simulink model "MAS"  (R2023a)
settings: Solver=FixedStepAuto  StartTime=0.0  StopTime=1  FixedStep=1e-6  RelTol=1e-5
values from neighbouring files (symbols this model uses):
  A_ob_w = [0, 0, 0, Msr*Rr/(rau*Ls*Lr) ... (first row only)    [main.m]
  A_observateur = [-Rsr/(rau*Ls), 0, Msr*Rr/(rau*Ls*Lr^2), 0 ... (first row only)    [main.m]
  abc_alpha_beta = sqrt(2/3) * [1, -1/2, -1/2 ... (first row only)    [main.m]
  B_observateur = [1/(rau*Ls),0 ... (first row only)    [main.m]
  Flux_1 = 1/(Msr^2 - Ls * Lr )  * [Rs*Lr, 0, -Rs*Msr, 0 ... (first row only)    [main.m]
  Flux_2 = 1/(Msr^2 - Ls * Lr )  * [0, 0, 0, 0 ... (first row only)    [main.m]
  frot = 0.01    [main.m]
  In = 8.3    [main.m]
  Inv_abc_alpha_beta = inv(abc_alpha_beta)    [main.m]
  Inv_Phi_Courant = inv(Phi_Courant)    [main.m]
  J = 0.025    [main.m]
  K_observateur = [-Rs/Ls-2*Pole, 0 ... (first row only)    [main.m]
  ki_reg_flux = K_reg_flux/T_reg_flux    (= 325705.222612)    [main.m]
  ki_reg_vitesse = K_reg_vitesse    (= 0.24)    [main.m]
  kid = ki/Ti    (= 11257.7319588)    [main.m]
  kiq = ki/Ti    (= 11257.7319588)    [main.m]
  kp_reg_flux = K_reg_flux    (= 179.885332059)    [main.m]
  kp_reg_vitesse = K_reg_vitesse/T_reg_vitesse    (= 0.625)    [main.m]
  kpd = ki    (= 19.9033319163)    [main.m]
  Kpi = ws*20    (= 6283.18530718)    [main.m]
  kpq = ki    (= 19.9033319163)    [main.m]
  Lr = 0.194    [main.m]
  Ls = 0.182    [main.m]
  Msr = 0.182    [main.m]
  onduleur = V_MLI/3*[2,-1,-1 ... (first row only)    [main.m]
  p = 2    [main.m]
  Pole = 1    [main.m]
  Rr = 1.15    [main.m]
  sigma = 1-Msr^2/(Ls*Lr)    (= 0.0618556701031)    [main.m]
  T_charge = 0    [main.m]
  T_MLI = 1/F_MLI    (= 0.0001)    [main.m]
  Tin = sqrt(10)/Kpi    [main.m]
  V_MLI = 540    [main.m]
  Vn = 220    [main.m]
  ws = 2*pi*Fn    (= 314.159265359)    [main.m]
libraries: hdlsllib x5, simulink_extras x4, simulink x1
settings Model: SimulationMode=accelerator  Creator=philippecasteres  LastModifiedBy=philippecasteres
settings SolverCC: ZeroCrossAlgorithm=Adaptive
settings DebuggingCC: IgnoredZcDiagnostic=none

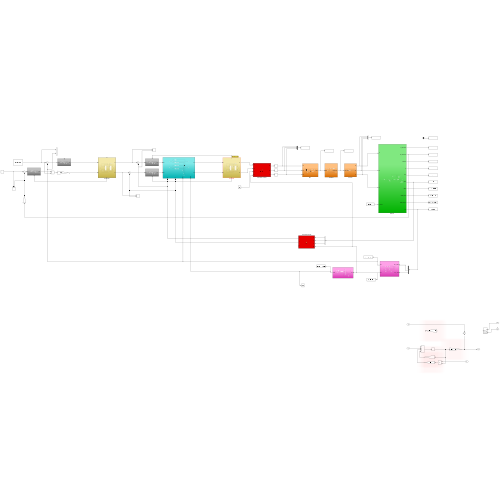
[thumbnail: Simulink's stored preview of the top-level diagram]
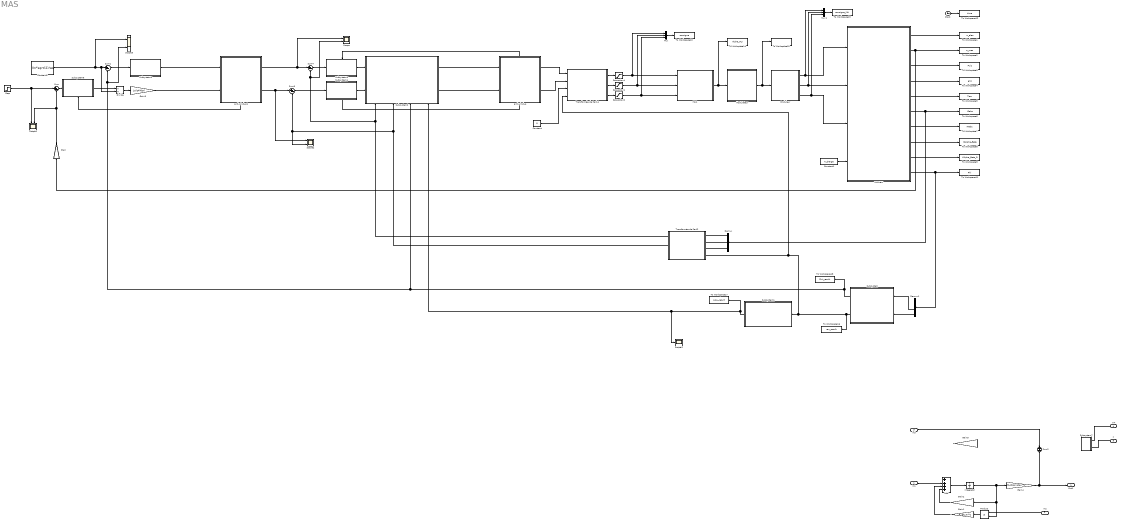
== system MAS ==
  In1 : Inport
  In2 : Inport  Port=2
  In3 : Inport  Port=3
  In4 : Inport  Port=4
  X : Inport  Port=5
  Add : Sum  Inputs=++++
  Clock : Clock
  Constant : Constant  Value=0
  Constant1 : Constant  Value=T_charge
  Constant2 : Constant  Value=Vn*sqrt(2)/ws
  Demux : Demux  Outputs=3
  Demux1 : Demux
  Divide : Product  Inputs=*/
  Gain : Gain  Gain=30/pi
  Gain1 : Gain  Gain=A_ob_w  Multiplication=Matrix(K*u)
  Gain2 : Gain  Gain=A_observateur  Multiplication=Matrix(K*u)
  Gain3 : Gain  Gain=Lr/(p*Msr)
  Gain4 : Gain  Gain=B_observateur  Multiplication=Matrix(K*u)
  Gain5 : Gain  Gain=K_observateur  Multiplication=Matrix(K*u)
  Integrator : Integrator
  MASnew : Subsystem
  MLI1 : Subsystem
  Modulateur : Subsystem
  Mux : Mux  Inputs=3
  Mux1 : Mux  Inputs=3
  Onduleur : Subsystem
  Product : Product
  Saturation1 : Saturate  UpperLimit=Vn*sqrt(2)  LowerLimit=-Vn*sqrt(2)
  Saturation2 : Saturate  UpperLimit=Vn*sqrt(2)  LowerLimit=-Vn*sqrt(2)
  Saturation4 : Saturate  UpperLimit=Vn*sqrt(2)  LowerLimit=-Vn*sqrt(2)
  Scope{,1..3} (4 alike) : Scope  NumInputPorts=2
  Scope4 : Scope
  Step : Step  Time=0.1  After=1450  SampleTime=0
  Subsystem : Subsystem
  Subsystem1 : Subsystem
  Subsystem2 : Subsystem
      settings: PortSchema="{\"entries\":[{\"content\":{\"sides\":[{\"content\":{\"connectorIds\":[\"In1\",\"In2\"]},\"type\":\"ConnectorPlacement.EquallySpacedRectSide\",\"uuid\":\"374a3029-9c19-44eb-9b98-de55e62c7022\"},{\"content\":{\"connectorIds\":[\"Out1\",\"Out2\"],\"side\":\"RIGHT\"},\"type\":\"ConnectorPlacement.EquallySpacedRectSide\",\"uuid\":\"b066ba17-ce68-41f6-a300-7d3bc4dc3f92\"},{\"content\":{\"side\":\"TOP\"},\"type\":\"ConnectorPlacement.EquallySpacedRectSide\",\"uuid\":\"ed738241-ae45-464d-a05c-a5861c3f77ca\"},{\"content\":{\"connectorIds\":[\"In3\",\"In4\",\"In5\",\"In6\"],\"side\":\"BOTTOM\"},\"type\":\"ConnectorPlacement.EquallySpacedRectSide\",\"uuid\":\"e5249242-5c32-4682-b932-0c2aba441929\"}]},\"type\":\"ConnectorPlacement.EquallySpacedConnector\",\"uuid\":\"519ae50f-d565-4f6e-aabe-7acf3d791e4a\"}],\"packageUris\":[\"http://schema.mathworks.com/mf0/Connector/R2020b\"],\"version\":\"1.0\"}"
  Subsystem3 : Subsystem
      settings: PortSchema="{\"entries\":[{\"content\":{\"sides\":[{\"content\":{\"connectorIds\":[\"In1\"]},\"type\":\"ConnectorPlacement.EquallySpacedRectSide\",\"uuid\":\"e479fa30-fafe-4b33-9f29-bcdfd025492c\"},{\"content\":{\"connectorIds\":[\"Out1\"],\"side\":\"RIGHT\"},\"type\":\"ConnectorPlacement.EquallySpacedRectSide\",\"uuid\":\"004bb801-1125-495b-9383-1b89d3712869\"},{\"content\":{\"connectorIds\":[\"In2\"],\"side\":\"TOP\"},\"type\":\"ConnectorPlacement.EquallySpacedRectSide\",\"uuid\":\"eb300401-215a-493c-865f-c89d4f0da9de\"}]},\"type\":\"ConnectorPlacement.EquallySpacedConnector\",\"uuid\":\"4261b941-699b-4a50-9a10-aa37cbe6dd2a\"}],\"packageUris\":[\"http://schema.mathworks.com/mf0/Connector/R2020b\"],\"version\":\"1.0\"}"
  Subsystem4 : Subsystem
      settings: PortSchema="{\"entries\":[{\"content\":{\"sides\":[{\"content\":{\"connectorIds\":[\"In1\"]},\"type\":\"ConnectorPlacement.EquallySpacedRectSide\",\"uuid\":\"b47c6917-9341-4daa-88c1-000b41eb9d38\"},{\"content\":{\"connectorIds\":[\"Out1\"],\"side\":\"RIGHT\"},\"type\":\"ConnectorPlacement.EquallySpacedRectSide\",\"uuid\":\"db977880-8c33-40fc-933d-e73e745919fc\"},{\"content\":{\"side\":\"TOP\"},\"type\":\"ConnectorPlacement.EquallySpacedRectSide\",\"uuid\":\"c60e1241-7377-4c09-9831-21e7b95cd727\"},{\"content\":{\"connectorIds\":[\"In2\"],\"side\":\"BOTTOM\"},\"type\":\"ConnectorPlacement.EquallySpacedRectSide\",\"uuid\":\"7267beab-c733-40aa-ba5e-a945633c6122\"}]},\"type\":\"ConnectorPlacement.EquallySpacedConnector\",\"uuid\":\"e7c74c67-79e5-4b53-bf68-91e77d655faf\"}],\"packageUris\":[\"http://schema.mathworks.com/mf0/Connector/R2020b\"],\"version\":\"1.0\"}"
  Subsystem5 : Subsystem
      settings: PortSchema="{\"entries\":[{\"content\":{\"sides\":[{\"content\":{\"connectorIds\":[\"In1\"]},\"type\":\"ConnectorPlacement.EquallySpacedRectSide\",\"uuid\":\"b47c6917-9341-4daa-88c1-000b41eb9d38\"},{\"content\":{\"connectorIds\":[\"Out1\"],\"side\":\"RIGHT\"},\"type\":\"ConnectorPlacement.EquallySpacedRectSide\",\"uuid\":\"db977880-8c33-40fc-933d-e73e745919fc\"},{\"content\":{\"connectorIds\":[\"In2\"],\"side\":\"TOP\"},\"type\":\"ConnectorPlacement.EquallySpacedRectSide\",\"uuid\":\"c60e1241-7377-4c09-9831-21e7b95cd727\"}]},\"type\":\"ConnectorPlacement.EquallySpacedConnector\",\"uuid\":\"e7c74c67-79e5-4b53-bf68-91e77d655faf\"}],\"packageUris\":[\"http://schema.mathworks.com/mf0/Connector/R2020b\"],\"version\":\"1.0\"}"
  Subsystem6 : Subsystem
      settings: PortSchema="{\"entries\":[{\"content\":{\"sides\":[{\"content\":{\"connectorIds\":[\"In1\"]},\"type\":\"ConnectorPlacement.EquallySpacedRectSide\",\"uuid\":\"b47c6917-9341-4daa-88c1-000b41eb9d38\"},{\"content\":{\"connectorIds\":[\"Out1\"],\"side\":\"RIGHT\"},\"type\":\"ConnectorPlacement.EquallySpacedRectSide\",\"uuid\":\"db977880-8c33-40fc-933d-e73e745919fc\"},{\"content\":{\"side\":\"TOP\"},\"type\":\"ConnectorPlacement.EquallySpacedRectSide\",\"uuid\":\"c60e1241-7377-4c09-9831-21e7b95cd727\"},{\"content\":{\"connectorIds\":[\"In2\"],\"side\":\"BOTTOM\"},\"type\":\"ConnectorPlacement.EquallySpacedRectSide\",\"uuid\":\"995178c3-5227-47fa-849d-7fc8f375b837\"}]},\"type\":\"ConnectorPlacement.EquallySpacedConnector\",\"uuid\":\"e7c74c67-79e5-4b53-bf68-91e77d655faf\"}],\"packageUris\":[\"http://schema.mathworks.com/mf0/Connector/R2020b\"],\"version\":\"1.0\"}"
  Subsystem7 : Subsystem
  Sum{,1,4..5} (4 alike) : Sum  Inputs=|+-
  Sum2 : Sum  Inputs=+|-
  To Workspace1 : ToWorkspace  VariableName=w_elec  SaveFormat=Timeseries  SampleTime=-1
  To Workspace10 : ToWorkspace  VariableName=consigne  SaveFormat=Timeseries  SampleTime=-1
  To Workspace11 : ToWorkspace  VariableName=Phi  SaveFormat=Timeseries  SampleTime=-1
  To Workspace12 : ToWorkspace  VariableName=time  SaveFormat=Timeseries  SampleTime=-1
  To Workspace13 : ToWorkspace  VariableName=consigne_MLI  SaveFormat=Timeseries  SampleTime=-1
  To Workspace14 : ToWorkspace  VariableName=Alpha_MLI  SaveFormat=Timeseries  SampleTime=-1
  To Workspace15 : ToWorkspace  VariableName=commande_Modulateur  SaveFormat=Timeseries  SampleTime=-1
  To Workspace16 : ToWorkspace  VariableName=rau_result  SaveFormat=Timeseries  SampleTime=-1
  To Workspace17 : ToWorkspace  VariableName=wrau_result  SaveFormat=Timeseries  SampleTime=-1
  To Workspace18 : ToWorkspace  VariableName=Phir_result  SaveFormat=Timeseries  SampleTime=-1
  To Workspace2 : ToWorkspace  VariableName=w_mec  SaveFormat=Timeseries  SampleTime=-1
  To Workspace3 : ToWorkspace  VariableName=Puis  SaveFormat=Timeseries  SampleTime=-1
  To Workspace4 : ToWorkspace  VariableName=glis  SaveFormat=Timeseries  SampleTime=-1
  To Workspace5 : ToWorkspace  VariableName=Tem  SaveFormat=Timeseries  SampleTime=-1
  To Workspace6 : ToWorkspace  VariableName=ISabc  SaveFormat=Timeseries  SampleTime=-1
  To Workspace7 : ToWorkspace  VariableName=IRabc  SaveFormat=Timeseries  SampleTime=-1
  To Workspace8 : ToWorkspace  VariableName=ISAlpha_Beta  SaveFormat=Timeseries  SampleTime=-1
  To Workspace9 : ToWorkspace  VariableName=VAlpha_Beta_O  SaveFormat=Timeseries  SampleTime=-1
  Transformée de Park-1 : MATLAB Function  TreatAsAtomicUnit=on
  Transformée de Park2 : MATLAB Function  TreatAsAtomicUnit=on
  anti-windup : Subsystem
      settings: PortSchema="{\"entries\":[{\"content\":{\"sides\":[{\"content\":{\"connectorIds\":[\"In1\",\"In2\"]},\"type\":\"ConnectorPlacement.EquallySpacedRectSide\",\"uuid\":\"233cb3cb-1249-40bd-bfdc-45fa9814c46e\"},{\"content\":{\"connectorIds\":[\"Out1\",\"Out2\"],\"side\":\"RIGHT\"},\"type\":\"ConnectorPlacement.EquallySpacedRectSide\",\"uuid\":\"0fdc860d-9a1f-453b-acef-69f40f5c198e\"},{\"content\":{\"connectorIds\":[\"Out4\"],\"side\":\"TOP\"},\"type\":\"ConnectorPlacement.EquallySpacedRectSide\",\"uuid\":\"10667f9d-69ec-4f3a-8ac8-5b780339c6a9\"},{\"content\":{\"connectorIds\":[\"Out3\"],\"side\":\"BOTTOM\"},\"type\":\"ConnectorPlacement.EquallySpacedRectSide\",\"uuid\":\"5505156d-5de0-4527-aff8-81b020aef34d\"}]},\"type\":\"ConnectorPlacement.EquallySpacedConnector\",\"uuid\":\"a7d416d1-7b5f-49c4-ac6f-32e00a36b461\"}],\"packageUris\":[\"http://schema.mathworks.com/mf0/Connector/R2020b\"],\"version\":\"1.0\"}"
  anti-windup1 : Subsystem
      settings: PortSchema="{\"entries\":[{\"content\":{\"sides\":[{\"content\":{\"connectorIds\":[\"In1\",\"In2\"]},\"type\":\"ConnectorPlacement.EquallySpacedRectSide\",\"uuid\":\"233cb3cb-1249-40bd-bfdc-45fa9814c46e\"},{\"content\":{\"connectorIds\":[\"Out1\",\"Out2\"],\"side\":\"RIGHT\"},\"type\":\"ConnectorPlacement.EquallySpacedRectSide\",\"uuid\":\"0fdc860d-9a1f-453b-acef-69f40f5c198e\"},{\"content\":{\"connectorIds\":[\"Out4\"],\"side\":\"TOP\"},\"type\":\"ConnectorPlacement.EquallySpacedRectSide\",\"uuid\":\"10667f9d-69ec-4f3a-8ac8-5b780339c6a9\"},{\"content\":{\"connectorIds\":[\"Out3\"],\"side\":\"BOTTOM\"},\"type\":\"ConnectorPlacement.EquallySpacedRectSide\",\"uuid\":\"5505156d-5de0-4527-aff8-81b020aef34d\"}]},\"type\":\"ConnectorPlacement.EquallySpacedConnector\",\"uuid\":\"a7d416d1-7b5f-49c4-ac6f-32e00a36b461\"}],\"packageUris\":[\"http://schema.mathworks.com/mf0/Connector/R2020b\"],\"version\":\"1.0\"}"
  Out1 : Outport
  wires:
  Onduleur/3(Vc) -> Mux1/3, MASnew/3(Vc)
  Transformée de Park-1/2(Vb) -> Saturation1/1
  MASnew/1(W_electrique) -> To Workspace1/1
  MASnew/3(puisance) -> To Workspace3/1
  MASnew/9(Valpha_beta_O) -> To Workspace9/1
  Subsystem3/1(Vd*) -> Subsystem2/1(Vd*)
  Demux1/4 -> Subsystem/2(Phi_r_beta)
  anti-windup/2(y1) -> Transformée de Park-1/2(Vq)
  MASnew/5(Tem) -> To Workspace5/1
  Modulateur/1(commande) -> To Workspace15/1, Onduleur/1(commande)
  Demux/1 -> Transformée de Park2/1(Ia)
  Subsystem1/1(Wrau) -> Scope4/1, Subsystem2/6(Wrau), To Workspace17/1
  Mux1/1 -> To Workspace13/1
  Constant/1 -> Transformée de Park-1/3(Vh)
  Saturation4/1 -> Mux/1, MLI1/1(Va*)
  Demux/3 -> Transformée de Park2/3(Ic)
  MASnew/4(g) -> To Workspace4/1
  Demux1/3 -> Subsystem/1(Phi_r_alpha)
  Transformée de Park2/1(Id) -> Scope/2, Sum4/2, Subsystem2/3(Id)
  Onduleur/1(Va) -> Mux1/1, MASnew/1(Va)
  Subsystem/1(Phir) -> To Workspace18/1, Scope3/2, Sum1/2, Subsystem2/5(Phir)
  MLI1/1(Alpha) -> To Workspace14/1, Modulateur/1(Alpha)
  Transformée de Park2/2(Iq) -> Sum5/2, Scope2/2, Subsystem2/4(Iq)
  Clock/1 -> To Workspace12/1
  Transformée de Park-1/3(Vc) -> Saturation2/1
  Mux/1 -> To Workspace10/1
  anti-windup/1(x1) -> Transformée de Park-1/1(Vd)
  Subsystem4/1(Vq*) -> Subsystem2/2(Vq*)
  MASnew/10(Phi) -> Demux1/1, To Workspace11/1
  Sum4/1 -> Subsystem3/1(Id*)
  MASnew/6(ISabc) -> Demux/1, To Workspace6/1
  Subsystem/2(rau) -> Subsystem1/1(rau), Transformée de Park-1/4(rau), Transformée de Park2/4(rau), To Workspace16/1
  Demux/2 -> Transformée de Park2/2(Ib)
  Onduleur/2(Vb) -> Mux1/2, MASnew/2(Vb)
  Saturation1/1 -> Mux/2, MLI1/2(Vb*)
  Sum5/1 -> Subsystem4/1(Iq*)
  Transformée de Park-1/1(Va) -> Saturation4/1
  MASnew/8(ISalpha_beta) -> To Workspace8/1
  Saturation2/1 -> Mux/3, MLI1/3(Vc*)
  MASnew/7(IRabc) -> To Workspace7/1
  Constant1/1 -> MASnew/4(T_charge)
  Divide/1 -> Gain3/1
  Sum1/1 -> Subsystem5/1(phir*)
  Subsystem6/1(Ce*) -> Divide/1
  Constant2/1 -> Scope3/1, Sum1/1, Divide/2
  Sum/1 -> Subsystem6/1(w*)
  Step/1 -> Sum/1, Scope1/1
  MASnew/2(W_mecanique) -> To Workspace2/1, Gain/1
  Gain/1 -> Scope1/2, Sum/2
  Gain3/1 -> anti-windup1/2(y)  "Iq"
  anti-windup1/2(y1) -> Scope2/1, Sum5/1
  anti-windup1/1(x1) -> Scope/1, Sum4/1
  Subsystem5/1(Id*) -> anti-windup1/1(x)
  Subsystem2/1(Vd) -> anti-windup/1(x)
  Subsystem2/2(Vq) -> anti-windup/2(y)
  anti-windup1/3(Out4) -> Subsystem6/2(u)
  anti-windup/4(u) -> Subsystem3/2(u)
  anti-windup/3(Out4) -> Subsystem4/2(u)
  Add/1 -> Integrator/1
  Product/1 -> Gain1/1
  In2/1 -> Product/1
  Integrator/1 -> Gain4/1, Gain2/1, Product/2
  Gain4/1 -> Out1/1, Sum2/2
  In3/1 -> Sum2/1
  Gain2/1 -> Add/4
  Gain1/1 -> Add/3
  In1/1 -> Add/2
  In4/1 -> Subsystem7/1(w)
  X/1 -> Subsystem7/2(X)

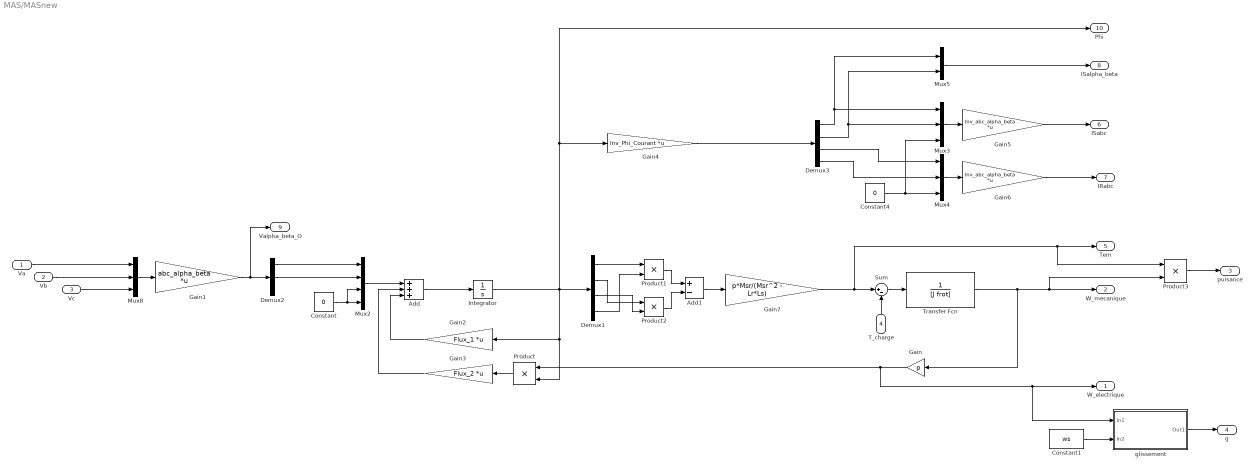
== system MAS/MASnew ==
  Va : Inport
  Vb : Inport  Port=2
  Vc : Inport  Port=3
  T_charge : Inport  Port=4
  Add : Sum  Inputs=+++
  Add1 : Sum  Inputs=+-
  Constant : Constant  Value=0
  Constant1 : Constant  Value=ws
  Constant4 : Constant  Value=0
  Demux1 : Demux
  Demux2 : Demux  Outputs=3
  Demux3 : Demux
  Gain : Gain  Gain=p
  Gain1 : Gain  Gain=abc_alpha_beta  Multiplication=Matrix(K*u)
  Gain2 : Gain  Gain=Flux_1  Multiplication=Matrix(K*u)
  Gain3 : Gain  Gain=Flux_2  Multiplication=Matrix(K*u)
  Gain4 : Gain  Gain=Inv_Phi_Courant  Multiplication=Matrix(K*u)
  Gain5 : Gain  Gain=Inv_abc_alpha_beta  Multiplication=Matrix(K*u)
  Gain6 : Gain  Gain=Inv_abc_alpha_beta  Multiplication=Matrix(K*u)
  Gain7 : Gain  Gain=p*Msr/(Msr^2 - Lr*Ls)
  Integrator : Integrator
  Mux2 : Mux
  Mux3 : Mux  Inputs=3
  Mux4 : Mux  Inputs=3
  Mux5 : Mux  Inputs=2
  Mux8 : Mux  Inputs=3
  Product{,1..3} (4 alike) : Product
  Sum : Sum  Inputs=|+-
  Transfer Fcn : TransferFcn  Denominator=[J frot]
  glissement : Subsystem
  W_electrique : Outport
  W_mecanique : Outport  Port=2
  puisance : Outport  Port=3
  g : Outport  Port=4
  Tem : Outport  Port=5
  ISabc : Outport  Port=6
  IRabc : Outport  Port=7
  ISalpha_beta : Outport  Port=8
  Valpha_beta_O : Outport  Port=9
  Phi : Outport  Port=10
  wires:
  Demux3/4 -> Mux4/2
  Demux3/2 -> Mux3/2, Mux5/2
  T_charge/1 -> Sum/2
  Demux3/1 -> Mux3/1, Mux5/1
  Va/1 -> Mux8/1
  Sum/1 -> Transfer Fcn/1
  Demux1/1 -> Product1/1
  Demux3/3 -> Mux4/1
  Gain7/1 -> Sum/1, Product3/1, Tem/1
  Transfer Fcn/1 -> Gain/1, Product3/2, W_mecanique/1
  Add/1 -> Integrator/1
  Vc/1 -> Mux8/3
  Vb/1 -> Mux8/2
  Product/1 -> Gain3/1
  Integrator/1 -> Gain2/1, Product/2, Demux1/1, Gain4/1, Phi/1
  Mux2/1 -> Add/1
  Mux3/1 -> Gain5/1
  Mux5/1 -> ISalpha_beta/1
  Gain1/1 -> Valpha_beta_O/1, Demux2/1
  Mux8/1 -> Gain1/1
  Demux2/1 -> Mux2/1
  Demux2/2 -> Mux2/2
  Constant/1 -> Mux2/4, Mux2/3
  Gain2/1 -> Add/3
  Gain4/1 -> Demux3/1
  Constant4/1 -> Mux4/3, Mux3/3
  Gain5/1 -> ISabc/1
  Mux4/1 -> Gain6/1
  Gain6/1 -> IRabc/1
  Product1/1 -> Add1/1
  Product2/1 -> Add1/2
  Add1/1 -> Gain7/1
  Gain/1 -> glissement/1(In1), W_electrique/1, Product/1
  Gain3/1 -> Add/2
  Demux1/4 -> Product1/2
  Demux1/2 -> Product2/1
  Demux1/3 -> Product2/2
  Product3/1 -> puisance/1
  glissement/1(Out1) -> g/1
  Constant1/1 -> glissement/2(In2)

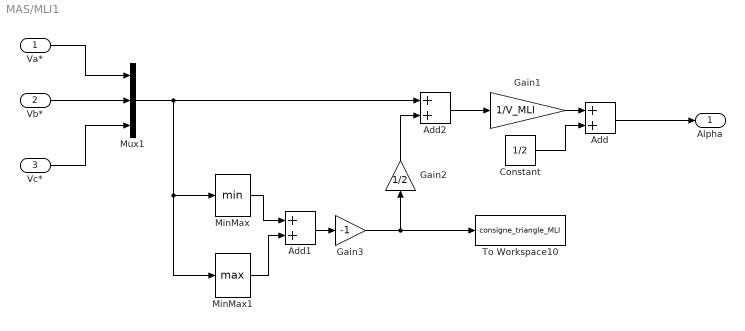
== system MAS/MLI1 ==
  Va* : Inport
  Vb* : Inport  Port=2
  Vc* : Inport  Port=3
  Add : Sum
  Add1 : Sum
  Add2 : Sum
  Constant : Constant  Value=1/2
  Gain1 : Gain  Gain=1/V_MLI
  Gain2 : Gain  Gain=1/2
  Gain3 : Gain  Gain=-1
  MinMax : MinMax
  MinMax1 : MinMax  Function=max
  Mux1 : Mux  Inputs=3
  To Workspace10 : ToWorkspace  VariableName=consigne_triangle_MLI  SaveFormat=Timeseries  SampleTime=-1
  Alpha : Outport
  wires:
  Va*/1 -> Mux1/1
  Gain1/1 -> Add/1
  Vb*/1 -> Mux1/2
  Vc*/1 -> Mux1/3
  Add/1 -> Alpha/1
  Add2/1 -> Gain1/1
  Constant/1 -> Add/2
  Gain2/1 -> Add2/2
  Mux1/1 -> Add2/1, MinMax/1, MinMax1/1
  Add1/1 -> Gain3/1
  MinMax/1 -> Add1/1
  MinMax1/1 -> Add1/2
  Gain3/1 -> To Workspace10/1, Gain2/1

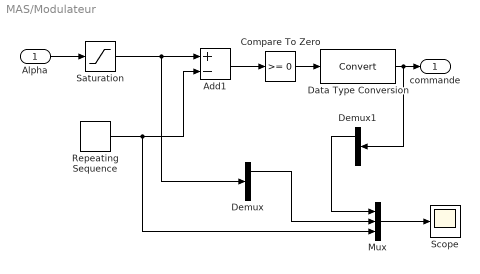
== system MAS/Modulateur ==
  Alpha : Inport
  Add1 : Sum  Inputs=+-
  Compare To Zero : hdlsllib/Logic and Bit Operations/Compare To Zero  relop=>=  OutDataTypeStr=boolean
  Data Type Conversion : DataTypeConversion  SaturateOnIntegerOverflow=off  RndMeth=Floor
  Demux : Demux  Outputs=3
  Demux1 : Demux  Outputs=3
  Mux : Mux  Inputs=3
  Repeating Sequence : simulink/Sources/Repeating Sequence  rep_seq_t=[0 0.5*T_MLI T_MLI]  rep_seq_y=[1 0 1]
  Saturation : Saturate  UpperLimit=1  LowerLimit=0
  Scope : Scope
  commande : Outport
  wires:
  Alpha/1 -> Saturation/1
  Repeating Sequence/1 -> Mux/3, Add1/2
  Add1/1 -> Compare To Zero/1
  Saturation/1 -> Demux/1, Add1/1
  Compare To Zero/1 -> Data Type Conversion/1
  Data Type Conversion/1 -> Demux1/1, commande/1
  Mux/1 -> Scope/1
  Demux1/1 -> Mux/1
  Demux/1 -> Mux/2

== system MAS/Onduleur ==
  commande : Inport
  Demux : Demux  Outputs=3
  Gain : Gain  Gain=onduleur  Multiplication=Matrix(K*u)
  Va : Outport
  Vb : Outport  Port=2
  Vc : Outport  Port=3
  wires:
  Gain/1 -> Demux/1
  commande/1 -> Gain/1
  Demux/3 -> Vc/1
  Demux/1 -> Va/1
  Demux/2 -> Vb/1

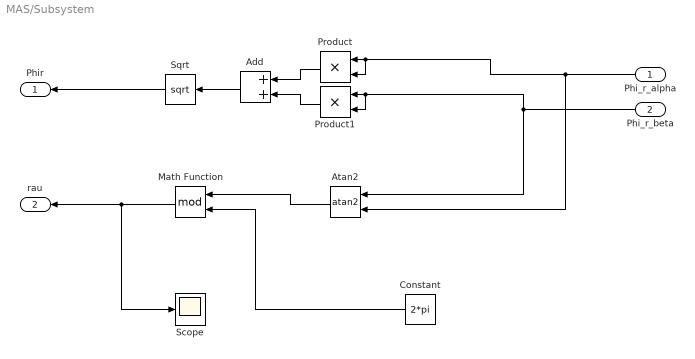
== system MAS/Subsystem ==
  Phi_r_alpha : Inport
  Phi_r_beta : Inport  Port=2
  Add : Sum
  Atan2 : Trigonometry  Operator=atan2
  Constant : Constant  Value=2*pi
  Math Function : Math  Operator=mod
  Product : Product
  Product1 : Product
  Scope : Scope
  Sqrt : Sqrt
  Phir : Outport
  rau : Outport  Port=2
  wires:
  Sqrt/1 -> Phir/1
  Product1/1 -> Add/2
  Add/1 -> Sqrt/1
  Phi_r_beta/1 -> Atan2/1, Product1/2, Product1/1
  Product/1 -> Add/1
  Phi_r_alpha/1 -> Atan2/2, Product/2, Product/1
  Atan2/1 -> Math Function/1
  Constant/1 -> Math Function/2
  Math Function/1 -> Scope/1, rau/1

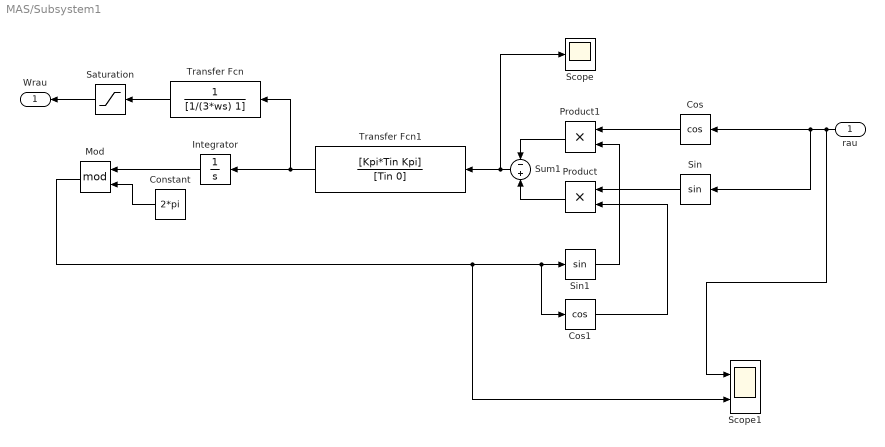
== system MAS/Subsystem1 ==
  rau : Inport
  Constant : Constant  Value=2*pi
  Cos : Trigonometry  Operator=cos
  Cos1 : Trigonometry  Operator=cos
  Integrator : Integrator
  Mod : Math  Operator=mod
  Product : Product
  Product1 : Product
  Saturation : Saturate  UpperLimit=2*ws  LowerLimit=-2*ws
  Scope : Scope
  Scope1 : Scope  NumInputPorts=2
  Sin : Trigonometry
  Sin1 : Trigonometry
  Sum1 : Sum  Inputs=-|+
  Transfer Fcn : TransferFcn  Denominator=[1/(3*ws) 1]
  Transfer Fcn1 : TransferFcn  Numerator=[Kpi*Tin Kpi]  Denominator=[Tin 0]
  Wrau : Outport
  wires:
  Constant/1 -> Mod/2
  Integrator/1 -> Mod/1
  Mod/1 -> Scope1/2, Cos1/1, Sin1/1
  Sum1/1 -> Scope/1, Transfer Fcn1/1
  rau/1 -> Scope1/1, Sin/1, Cos/1
  Sin/1 -> Product/1
  Cos/1 -> Product1/1
  Sin1/1 -> Product1/2
  Cos1/1 -> Product/2
  Product1/1 -> Sum1/1
  Product/1 -> Sum1/2
  Transfer Fcn/1 -> Saturation/1
  Transfer Fcn1/1 -> Transfer Fcn/1, Integrator/1
  Saturation/1 -> Wrau/1

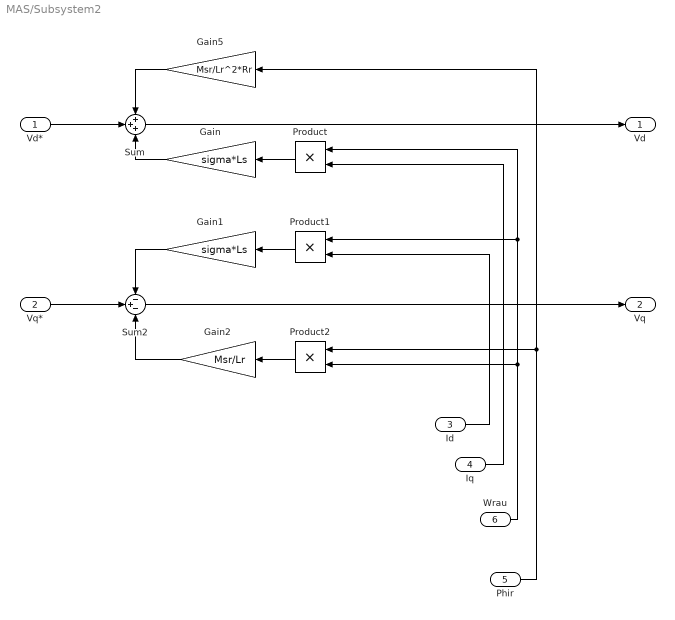
== system MAS/Subsystem2 ==
  Vd* : Inport
  Vq* : Inport  Port=2
  Id : Inport  Port=3
  Iq : Inport  Port=4
  Phir : Inport  Port=5
  Wrau : Inport  Port=6
  Gain : Gain  Gain=sigma*Ls
  Gain1 : Gain  Gain=sigma*Ls
  Gain2 : Gain  Gain=Msr/Lr
  Gain5 : Gain  Gain=Msr/Lr^2*Rr
  Product : Product
  Product1 : Product
  Product2 : Product
  Sum : Sum  Inputs=+++
  Sum2 : Sum  Inputs=-+-
  Vd : Outport
  Vq : Outport  Port=2
  wires:
  Vd*/1 -> Sum/2
  Iq/1 -> Product/2
  Id/1 -> Product1/2
  Gain/1 -> Sum/3
  Product/1 -> Gain/1
  Gain1/1 -> Sum2/1
  Product1/1 -> Gain1/1
  Vq*/1 -> Sum2/2
  Wrau/1 -> Product2/2, Product1/1, Product/1
  Phir/1 -> Product2/1, Gain5/1
  Gain5/1 -> Sum/1
  Sum2/1 -> Vq/1
  Product2/1 -> Gain2/1
  Sum/1 -> Vd/1
  Gain2/1 -> Sum2/3

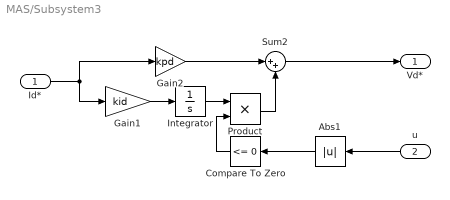
== system MAS/Subsystem3 ==
  Id* : Inport
  u : Inport  Port=2
  Abs1 : Abs  SaturateOnIntegerOverflow=off
  Compare To Zero : hdlsllib/Logic and Bit Operations/Compare To Zero  relop=<=  OutDataTypeStr=boolean
  Gain1 : Gain  Gain=kid
  Gain2 : Gain  Gain=kpd
  Integrator : Integrator
  Product : Product
  Sum2 : Sum  Inputs=|++
  Vd* : Outport
  wires:
  Gain1/1 -> Integrator/1
  Integrator/1 -> Product/1
  Compare To Zero/1 -> Product/2
  Id*/1 -> Gain1/1, Gain2/1
  Product/1 -> Sum2/2
  Sum2/1 -> Vd*/1
  u/1 -> Abs1/1
  Abs1/1 -> Compare To Zero/1
  Gain2/1 -> Sum2/1

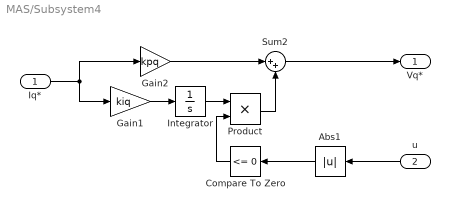
== system MAS/Subsystem4 ==
  Iq* : Inport
  u : Inport  Port=2
  Abs1 : Abs  SaturateOnIntegerOverflow=off
  Compare To Zero : hdlsllib/Logic and Bit Operations/Compare To Zero  relop=<=  OutDataTypeStr=boolean
  Gain1 : Gain  Gain=kiq
  Gain2 : Gain  Gain=kpq
  Integrator : Integrator
  Product : Product
  Sum2 : Sum  Inputs=|++
  Vq* : Outport
  wires:
  Gain1/1 -> Integrator/1
  Integrator/1 -> Product/1
  Iq*/1 -> Gain1/1, Gain2/1
  Product/1 -> Sum2/2
  Sum2/1 -> Vq*/1
  Compare To Zero/1 -> Product/2
  Abs1/1 -> Compare To Zero/1
  u/1 -> Abs1/1
  Gain2/1 -> Sum2/1

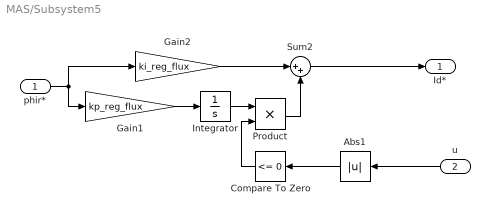
== system MAS/Subsystem5 ==
  phir* : Inport
  u : Inport  Port=2
  Abs1 : Abs  SaturateOnIntegerOverflow=off
  Compare To Zero : hdlsllib/Logic and Bit Operations/Compare To Zero  relop=<=  OutDataTypeStr=boolean
  Gain1 : Gain  Gain=kp_reg_flux
  Gain2 : Gain  Gain=ki_reg_flux
  Integrator : Integrator
  Product : Product
  Sum2 : Sum  Inputs=|++
  Id* : Outport
  wires:
  Gain1/1 -> Integrator/1
  Integrator/1 -> Product/1
  Compare To Zero/1 -> Product/2
  phir*/1 -> Gain2/1, Gain1/1
  Product/1 -> Sum2/2
  Sum2/1 -> Id*/1
  Abs1/1 -> Compare To Zero/1
  u/1 -> Abs1/1
  Gain2/1 -> Sum2/1

== system MAS/Subsystem6 ==
  w* : Inport
  u : Inport  Port=2
  Abs1 : Abs  SaturateOnIntegerOverflow=off
  Compare To Zero : hdlsllib/Logic and Bit Operations/Compare To Zero  relop=<=  OutDataTypeStr=boolean
  Gain1 : Gain  Gain=ki_reg_vitesse
  Gain2 : Gain  Gain=kp_reg_vitesse
  Integrator : Integrator
  Product : Product
  Sum2 : Sum  Inputs=|++
  Ce* : Outport
  wires:
  Gain1/1 -> Integrator/1
  Integrator/1 -> Product/1
  w*/1 -> Gain1/1, Gain2/1
  Product/1 -> Sum2/2
  Sum2/1 -> Ce*/1
  Compare To Zero/1 -> Product/2
  Abs1/1 -> Compare To Zero/1
  u/1 -> Abs1/1
  Gain2/1 -> Sum2/1

== system MAS/Subsystem7 ==
  w : Inport
  X : Inport  Port=2
  Constant3 : Constant  Value=Pole
  Constant4 : Constant  Value=Ls
  MATLAB Function : MATLAB Function  TreatAsAtomicUnit=on
  K_w : Outport
  wires:
  MATLAB Function/1(K_w) -> K_w/1
  X/1 -> MATLAB Function/1(X)
  Constant4/1 -> MATLAB Function/3(Ls)
  w/1 -> MATLAB Function/2(w)
  Constant3/1 -> MATLAB Function/4(Pole)

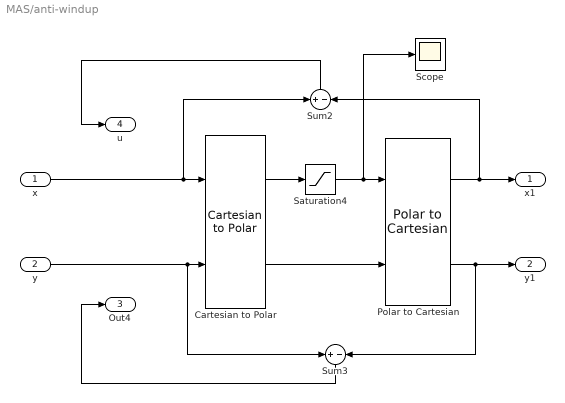
== system MAS/anti-windup ==
  x : Inport
  y : Inport  Port=2
  Cartesian to Polar : simulink_extras/Transformations/Cartesian to Polar
  Polar to Cartesian : simulink_extras/Transformations/Polar to Cartesian
  Saturation4 : Saturate  UpperLimit=V_MLI/sqrt(3)  LowerLimit=0
  Scope : Scope
  Sum2 : Sum  Inputs=+|-
  Sum3 : Sum  Inputs=+|-
  x1 : Outport
  y1 : Outport  Port=2
  Out4 : Outport  Port=3
  u : Outport  Port=4
  wires:
  Polar to Cartesian/2 -> Sum3/2, y1/1
  Polar to Cartesian/1 -> Sum2/2, x1/1
  x/1 -> Sum2/1, Cartesian to Polar/1
  Sum2/1 -> u/1
  y/1 -> Sum3/1, Cartesian to Polar/2
  Cartesian to Polar/1 -> Saturation4/1
  Cartesian to Polar/2 -> Polar to Cartesian/2
  Sum3/1 -> Out4/1
  Saturation4/1 -> Scope/1, Polar to Cartesian/1

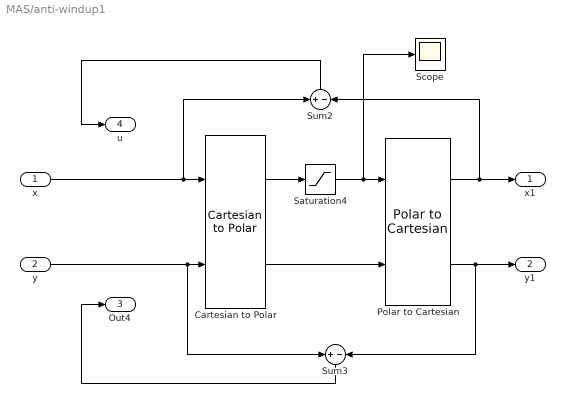
== system MAS/anti-windup1 ==
  x : Inport
  y : Inport  Port=2
  Cartesian to Polar : simulink_extras/Transformations/Cartesian to Polar
  Polar to Cartesian : simulink_extras/Transformations/Polar to Cartesian
  Saturation4 : Saturate  UpperLimit=2*In  LowerLimit=0
  Scope : Scope
  Sum2 : Sum  Inputs=+|-
  Sum3 : Sum  Inputs=+|-
  x1 : Outport
  y1 : Outport  Port=2
  Out4 : Outport  Port=3
  u : Outport  Port=4
  wires:
  Polar to Cartesian/2 -> Sum3/2, y1/1
  Polar to Cartesian/1 -> Sum2/2, x1/1
  x/1 -> Sum2/1, Cartesian to Polar/1
  Sum2/1 -> u/1
  y/1 -> Sum3/1, Cartesian to Polar/2
  Cartesian to Polar/1 -> Saturation4/1
  Cartesian to Polar/2 -> Polar to Cartesian/2
  Sum3/1 -> Out4/1
  Saturation4/1 -> Scope/1, Polar to Cartesian/1

== system MAS/MASnew/glissement ==
  In1 : Inport
  In2 : Inport  Port=2
  Add2 : Sum  Inputs=+-
  Divide : Product  Inputs=*/
  Out1 : Outport
  wires:
  In2/1 -> Divide/2, Add2/1
  Divide/1 -> Out1/1
  In1/1 -> Add2/2
  Add2/1 -> Divide/1

== matlab function MAS/Transformée de Park-1 ==
  data: Vd input; Va output; Vb output; Vc output; Vq input; Vh input; rau input
function [Va, Vb, Vc] = dq_abc(Vd,Vq,Vh,rau)


    % Vecteur de tensions d'entrée
    V = [Vd;Vq;Vh];
    
    % Matrice de transformation
    transformation_matrix = sqrt(2/3)*[cos(rau), cos(rau - 2*pi/3), cos(rau + 2*pi/3);
                                         -sin(rau), -sin(rau - 2*pi/3), -sin(rau + 2*pi/3);
                                          1/sqrt(2), 1/sqrt(2), 1/sqrt(2)];
    
    % Calcul des résultats
    result = inv(transformation_matrix) * V;
    
    % Attribution des résultats aux sorties
    Va = result(1);
    Vb= result(2);
    Vc = result(3);




end

== matlab function MAS/Subsystem7/MATLAB Function ==
  data: X input; w input; K_w output; Ls input; Pole input
function K_w = Kw(X,w,Ls,Pole)



L = [0, w;
        w,0;
        Ls*w^2, 2*Ls*w*Pole;
        -2*Ls*w*Pole,Ls*w^2];
K_w=L.*X;
end

== matlab function MAS/Transformée de Park2 ==
  data: Ia input; Id output; Iq output; Ih output; Ib input; Ic input; rau input
function [Id,Iq,Ih] = abc_dq(Ia, Ib, Ic,rau)


    % Vecteur de tensions d'entrée
    I = [Ia; Ib; Ic];
    
    % Matrice de transformation
    transformation_matrix =sqrt(2/3)*[cos(rau), cos(rau - 2*pi/3), cos(rau + 2*pi/3);
                                         -sin(rau), -sin(rau - 2*pi/3), -sin(rau + 2*pi/3);
                                          1/sqrt(2), 1/sqrt(2), 1/sqrt(2)];
    
    % Calcul des résultats
    result = transformation_matrix * I;
    
    % Attribution des résultats aux sorties
    Id = result(1);
    Iq= result(2);
    Ih = result(3);




end
